simulink model "MultiAgentQUAV"  (R2017a)
settings: Solver=ode1  StartTime=0.0  StopTime=50  FixedStep=tstep  RelTol=1e-3
InitFcn:
  | initSim;
StopFcn:
  | plotSimSolution;
values from neighbouring files (symbols this model uses):
  N = cross(u,v)'    [MultiAgentQUAVPlantNewtOLD.m]    (also in MultiAgentQUAVProblemNewt.m = size(phi,1); initSim.m = 20)
  tstep = 0.1    [initSim.m]
undefined symbols (not defined in the file or in its folder): m, problem, X, Y, Z
libraries: nesl_utility x38, sm_lib x25, sharedtransform x4
(part 3 of 3)

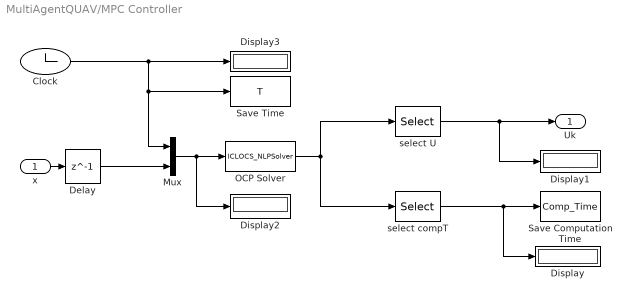
== system MultiAgentQUAV/MPC Controller  ==
  x : Inport
  Clock : Clock
  Delay : Delay  DelayLength=1  InitialCondition=[problem.states.x0]
  Display{,1..3} (4 alike) : Display
  Mux : Mux  Inputs=2
  OCP Solver : MATLABFcn  MATLABFcn=ICLOCS_NLPSolver  OutputDimensions=m+2
  "Save Computation Time " : ToWorkspace  VariableName=Comp_Time  SampleTime=tstep
      settings: Save2DSignal=2-D array (concatenate along first dimension)
  Save Time : ToWorkspace  VariableName=T  SampleTime=-1
      settings: Save2DSignal=2-D array (concatenate along first dimension)
  select U : Selector  IndexOptions=Index vector (dialog)  Indices=3:m+2  OutputSizes=1
  select compT : Selector  IndexOptions=Index vector (dialog)  Indices=2  OutputSizes=1
  Uk : Outport
  wires:
  select U/1 -> Display1/1, Uk/1
  x/1 -> Delay/1
  OCP Solver/1 -> select U/1, select compT/1
  Clock/1 -> Save Time/1, Mux/1, Display3/1
  select compT/1 -> Display/1, "Save Computation Time "/1
  Mux/1 -> Display2/1, OCP Solver/1
  Delay/1 -> Mux/2
